simulink model "NoiseGen"  (R2016a)
settings: Solver=VariableStepAuto  StartTime=0.0  StopTime=1000  RelTol=1e-3
InitFcn:
  | LFSR=16
  | Ts=3/280e6
libraries: xbsIndex_r4 x31
settings Model: Creator=frank  LastModifiedBy=frank

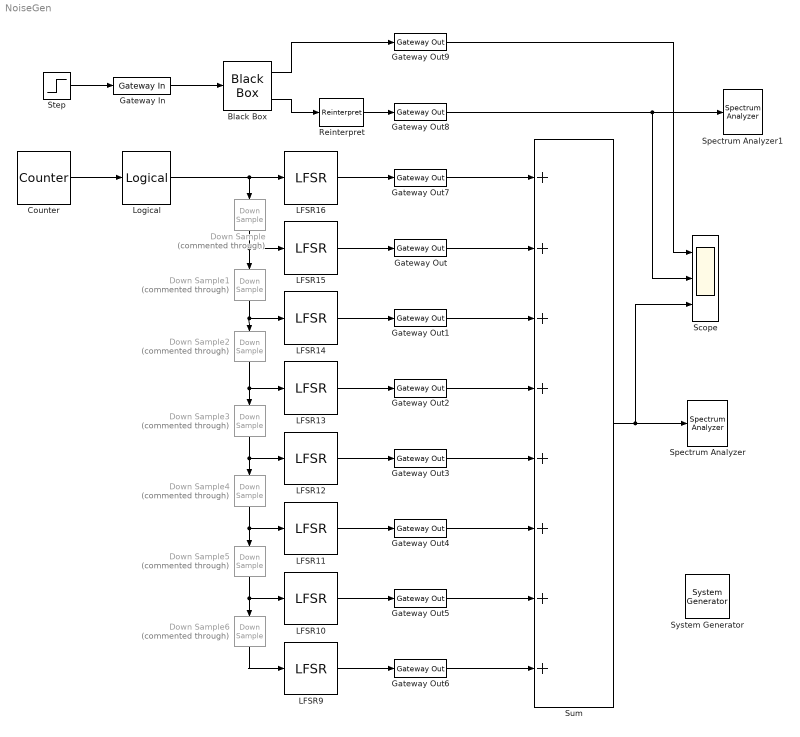
== system NoiseGen ==
  " System Generator" : xbsIndex_r4/ System Generator  Tag=genX  xilinxfamily=kintex7  part=xc7k325t  speed=-2  package=fbg676  synthesis_tool=Vivado  clock_wrapper=Clock Enables  directory=./netlist  proj_type=Vivado  Synth_file=Vivado Synthesis Defaults  Impl_file=Vivado Implementation Defaults  testbench=off  simulink_period=Ts  sysclk_period=10  dcm_input_clock_period=10  incr_netlist=off  trim_vbits=Everywhere in SubSystem  dbl_ovrd=According to Block Masks  core_generation=According to Block Masks  run_coregen=off  deprecated_control=off  eval_field=0  block_type=sysgen
  Black Box : xbsIndex_r4/Black Box  init_code=gng_config  sim_method=ISE Simulator  verbose=off  block_type=blackbox2
  Counter : xbsIndex_r4/Counter  cnt_type=Count Limited  cnt_to=4  operation=Up  start_count=0  cnt_by_val=1  arith_type=Unsigned  n_bits=8  bin_pt=0  load_pin=off  rst=off  en=off  explicit_period=on  period=Ts  use_behavioral_HDL=off  implementation=Fabric  dbl_ovrd=off  block_type=counter
  Down Sample{,1..6} (7 alike) : xbsIndex_r4/Down Sample  Commented=through  sample_ratio=2  sample_phase="Last Value of Frame  (most efficient)"  en=off  rst=off  latency=1  dbl_ovrd=off  block_type=dsamp
  Gateway In : xbsIndex_r4/Gateway In  gui_display_data_type=Boolean  arith_type=Boolean  n_bits=16  bin_pt=14  preci_type=Single  exp_width=8  frac_width=24  rows=1  columns=1  quantization="Round  (unbiased: +/- Inf)"  overflow=Saturate  period=Ts  UseAsADC=off  ADCChannel='1'  interface=None  automatic_assignment=on  address_offset=hex2dec('00')  intf_name=''  intf_description=''  default_value=0  timing_constraint=None  locs_specified=off  LOCs={}  io_standard={}  inherit_from_input=off  hdl_port=on  dbl_ovrd=off  block_type=gatewayin
  Gateway Out{,1..9} (10 alike) : xbsIndex_r4/Gateway Out  inherit_from_input=off  hdl_port=on  rows=1  columns=1  UseAsDAC=off  DACChannel='1'  interface=None  automatic_assignment=on  address_offset=hex2dec('00')  intf_name=''  intf_description=''  timing_constraint=None  locs_specified=off  LOCs={}  io_standard={}  block_type=gatewayout
  LFSR10 : xbsIndex_r4/LFSR  lfsr_type=Fibonacci  gate_type=XNOR  n_bits=10  maxpolynomial=on  polynomial='121'  rst_value='3F'  rst=off  en=on  reloadable_seed=off  input_type=off  output_type=on  arith_type="Signed  (2's comp)"  bin_pt=9  explicit_period=off  period=1  dbl_ovrd=off  block_type=lfsr
  LFSR11 : xbsIndex_r4/LFSR  lfsr_type=Fibonacci  gate_type=XNOR  n_bits=11  maxpolynomial=on  polynomial='281'  rst_value='3F'  rst=off  en=on  reloadable_seed=off  input_type=off  output_type=on  arith_type="Signed  (2's comp)"  bin_pt=10  explicit_period=off  period=1  dbl_ovrd=off  block_type=lfsr
  LFSR12 : xbsIndex_r4/LFSR  lfsr_type=Fibonacci  gate_type=XNOR  n_bits=12  maxpolynomial=on  polynomial='415'  rst_value='3F'  rst=off  en=on  reloadable_seed=off  input_type=off  output_type=on  arith_type="Signed  (2's comp)"  bin_pt=11  explicit_period=off  period=1  dbl_ovrd=off  block_type=lfsr
  LFSR13 : xbsIndex_r4/LFSR  lfsr_type=Fibonacci  gate_type=XNOR  n_bits=13  maxpolynomial=on  polynomial='0807'  rst_value='3F'  rst=off  en=on  reloadable_seed=off  input_type=off  output_type=on  arith_type="Signed  (2's comp)"  bin_pt=12  explicit_period=off  period=1  dbl_ovrd=off  block_type=lfsr
  LFSR14 : xbsIndex_r4/LFSR  lfsr_type=Fibonacci  gate_type=XNOR  n_bits=14  maxpolynomial=on  polynomial='100b'  rst_value='3F'  rst=off  en=on  reloadable_seed=off  input_type=off  output_type=on  arith_type="Signed  (2's comp)"  bin_pt=13  explicit_period=off  period=1  dbl_ovrd=off  block_type=lfsr
  LFSR15 : xbsIndex_r4/LFSR  lfsr_type=Fibonacci  gate_type=XNOR  n_bits=15  maxpolynomial=on  polynomial='3001'  rst_value='3F'  rst=off  en=on  reloadable_seed=off  input_type=off  output_type=on  arith_type="Signed  (2's comp)"  bin_pt=14  explicit_period=off  period=1  dbl_ovrd=off  block_type=lfsr
  LFSR16 : xbsIndex_r4/LFSR  lfsr_type=Fibonacci  gate_type=XNOR  n_bits=16  maxpolynomial=on  polynomial='6805'  rst_value='3F'  rst=off  en=on  reloadable_seed=off  input_type=off  output_type=on  arith_type="Signed  (2's comp)"  bin_pt=15  explicit_period=off  period=1  dbl_ovrd=off  block_type=lfsr
  LFSR9 : xbsIndex_r4/LFSR  lfsr_type=Fibonacci  gate_type=XNOR  n_bits=9  maxpolynomial=on  polynomial='089'  rst_value='3F'  rst=off  en=on  reloadable_seed=off  input_type=off  output_type=on  arith_type="Signed  (2's comp)"  bin_pt=8  explicit_period=off  period=1  dbl_ovrd=off  block_type=lfsr
  Logical : xbsIndex_r4/Logical  logical_function=NOR  inputs=1  en=off  latency=1  precision=Full  arith_type=Unsigned  n_bits=16  bin_pt=0  align_bp=on  dbl_ovrd=off  block_type=logical
  Reinterpret : xbsIndex_r4/Reinterpret  force_arith_type=on  arith_type="Signed  (2's comp)"  force_bin_pt=on  bin_pt=15  block_type=reinterpret
  Scope : Scope  NumInputPorts=3
  Spectrum Analyzer : SpectrumAnalyzer
  Spectrum Analyzer1 : SpectrumAnalyzer
  Step : Step  Time=10*Ts  SampleTime=Ts
  Sum : Sum  Inputs=++++++++
  wires:
  LFSR15/1 -> Gateway Out/1
  Gateway Out/1 -> Sum/2
  Sum/1 -> Scope/3, Spectrum Analyzer/1
  LFSR14/1 -> Gateway Out1/1
  Gateway Out1/1 -> Sum/3
  LFSR13/1 -> Gateway Out2/1
  LFSR12/1 -> Gateway Out3/1
  Gateway Out2/1 -> Sum/4
  Gateway Out3/1 -> Sum/5
  LFSR11/1 -> Gateway Out4/1
  LFSR10/1 -> Gateway Out5/1
  LFSR9/1 -> Gateway Out6/1
  LFSR16/1 -> Gateway Out7/1
  Gateway Out7/1 -> Sum/1
  Gateway Out5/1 -> Sum/7
  Gateway Out6/1 -> Sum/8
  Gateway Out4/1 -> Sum/6
  Down Sample/1 -> Down Sample1/1, LFSR15/1
  Down Sample1/1 -> Down Sample2/1, LFSR14/1
  Down Sample2/1 -> Down Sample3/1, LFSR13/1
  Down Sample3/1 -> Down Sample4/1, LFSR12/1
  Down Sample4/1 -> Down Sample5/1, LFSR11/1
  Down Sample5/1 -> Down Sample6/1, LFSR10/1
  Down Sample6/1 -> LFSR9/1
  Logical/1 -> LFSR16/1, Down Sample/1
  Counter/1 -> Logical/1
  Gateway Out8/1 -> Spectrum Analyzer1/1, Scope/2
  Gateway Out9/1 -> Scope/1
  Black Box/1 -> Gateway Out9/1
  Black Box/2 -> Reinterpret/1
  Gateway In/1 -> Black Box/1
  Step/1 -> Gateway In/1
  Reinterpret/1 -> Gateway Out8/1
